simulink model "RedPrueba"  (R2015a)
settings: Solver=ode45  StartTime=0.0  StopTime=0.160  RelTol=1e-3
libraries: powerlib x20
settings Model: Creator=NECSOFT  LastModifiedBy=USUARIO

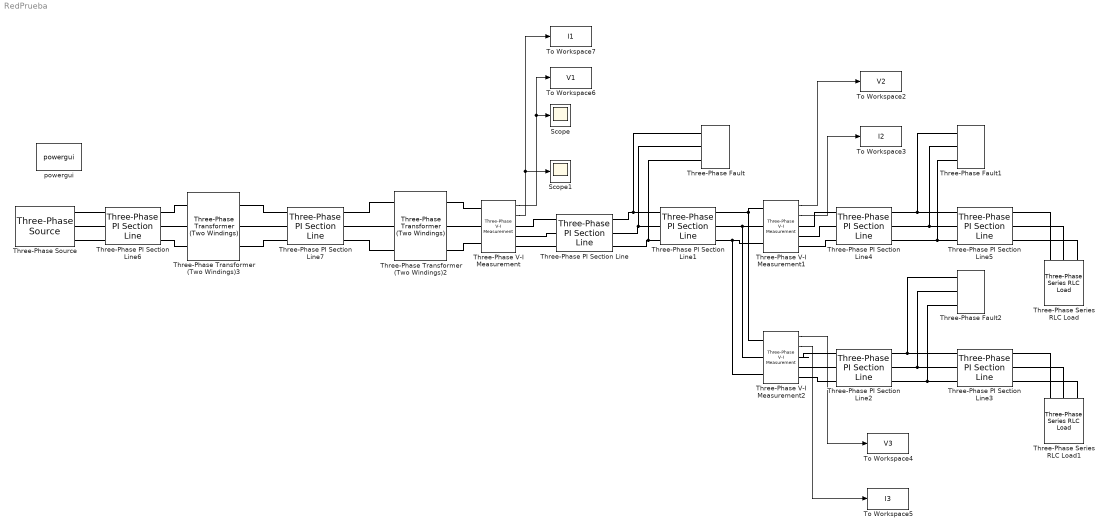
== system RedPrueba ==
  Scope : Scope
  Scope1 : Scope
  Three-Phase PI Section Line : powerlib/Elements/Three-Phase PI Section Line  LConnTagsString=a|b|c  RConnTagsString=A|B|C  Frequency=60  Resistances=[ 0.01273 0.3864]  Inductances="[ 0.9337e-3  4.1264e-3]"  Capacitances=[12.74e-9 7.751e-9]  Length=15
  Three-Phase PI Section Line1 : powerlib/Elements/Three-Phase PI Section Line  LConnTagsString=a|b|c  RConnTagsString=A|B|C  Frequency=60  Resistances=[ 0.01273 0.3864]  Inductances="[ 0.9337e-3  4.1264e-3]"  Capacitances=[12.74e-9 7.751e-9]  Length=5
  Three-Phase PI Section Line2 : powerlib/Elements/Three-Phase PI Section Line  LConnTagsString=a|b|c  RConnTagsString=A|B|C  Frequency=60  Resistances=[ 4*0.01273 4*0.3864]  Inductances="[ 4*0.9337e-3  4*4.1264e-3]"  Capacitances=[12.74e-9 7.751e-9]  Length=12
  Three-Phase PI Section Line3 : powerlib/Elements/Three-Phase PI Section Line  LConnTagsString=a|b|c  RConnTagsString=A|B|C  Frequency=60  Resistances=[ 4*0.01273 4*0.3864]  Inductances="[ 4*0.9337e-3  4*4.1264e-3]"  Capacitances=[12.74e-9 7.751e-9]  Length=8
  Three-Phase PI Section Line4 : powerlib/Elements/Three-Phase PI Section Line  LConnTagsString=a|b|c  RConnTagsString=A|B|C  Frequency=60  Resistances=[ 2*0.01273 2*0.3864]  Inductances="[ 2*0.9337e-3  2*4.1264e-3]"  Capacitances=[12.74e-9 7.751e-9]  Length=0.1
  Three-Phase PI Section Line5 : powerlib/Elements/Three-Phase PI Section Line  LConnTagsString=a|b|c  RConnTagsString=A|B|C  Frequency=60  Resistances=[ 2*0.01273 2*0.3864]  Inductances="[ 2*0.9337e-3  2*4.1264e-3]"  Capacitances=[12.74e-9 7.751e-9]  Length=19.9
  Three-Phase PI Section Line6 : powerlib/Elements/Three-Phase PI Section Line  LConnTagsString=a|b|c  RConnTagsString=A|B|C  Frequency=60  Resistances=[ 0.01273 0.3864]  Inductances="[ 0.9337e-3  4.1264e-3]"  Capacitances=[12.74e-9 7.751e-9]  Length=50
  Three-Phase PI Section Line7 : powerlib/Elements/Three-Phase PI Section Line  LConnTagsString=a|b|c  RConnTagsString=A|B|C  Frequency=60  Resistances=[ 0.01273 0.3864]  Inductances="[ 0.9337e-3  4.1264e-3]"  Capacitances=[12.74e-9 7.751e-9]  Length=100
  Three-Phase Series RLC Load : powerlib/Elements/Three-Phase Series RLC Load  LConnTagsString=A|B|C  Configuration=Y (grounded)  NominalVoltage=13800  NominalFrequency=60  ActivePower=100e3  InductivePower=0  CapacitivePower=0  Measurements=None  LoadType=constant Z
  Three-Phase Series RLC Load1 : powerlib/Elements/Three-Phase Series RLC Load  LConnTagsString=A|B|C  Configuration=Y (grounded)  NominalVoltage=13800  NominalFrequency=60  ActivePower=100e3  InductivePower=0  CapacitivePower=0  Measurements=None  LoadType=constant Z
  Three-Phase Transformer (Two Windings)2 : powerlib/Elements/Three-Phase Transformer (Two Windings)  Winding1Connection=Yg  Winding2Connection=Yg  CoreType=Three single-phase transformers  SetSaturation=off  Hysteresis=off  DataFile='hysteresis'  SetInitialFlux=off  Measurements=None  UNITS=pu  NominalPower=[ 5e6 , 60 ]  Winding1=[ 34500 , 0 , 0.0273 ]  Winding2=[ 13800 , 0 , 0.0273 ]  Rm=500  Lm=500  L0=0.5  Saturation=[ 0,0 ; 0.0024,1.2 ; 1.0,1.52 ]  InitialFluxes=[ 0.8 , -0.8 , 0.7 ]  MoreParameters=off  BreakLoop=off  DataType=off  TransfoNumber=1
  Three-Phase Transformer (Two Windings)3 : powerlib/Elements/Three-Phase Transformer (Two Windings)  Winding1Connection=Yg  Winding2Connection=Yg  CoreType=Three single-phase transformers  SetSaturation=off  Hysteresis=off  DataFile='hysteresis'  SetInitialFlux=off  Measurements=None  UNITS=pu  NominalPower=[ 40e6 , 60 ]  Winding1=[ 115000 , 0 , 0.06 ]  Winding2=[ 34500 , 0 , 0.06 ]  Rm=500  Lm=500  L0=0.5  Saturation=[ 0,0 ; 0.0024,1.2 ; 1.0,1.52 ]  InitialFluxes=[ 0.8 , -0.8 , 0.7 ]  MoreParameters=off  BreakLoop=off  DataType=off  TransfoNumber=1
  Three-Phase V-I Measurement : powerlib/Measurements/Three-Phase V-I Measurement  VoltageMeasurement=phase-to-ground  SetLabelV=off  LabelV=Vabc  Vpu=off  VpuLL=off  CurrentMeasurement=yes  SetLabelI=off  LabelI=Iabc  Ipu=off  Pbase=100e6  Vbase=500e3  OutputType=Complex  PhasorSimulation=off  PSBequivalent=0
  Three-Phase V-I Measurement1 : powerlib/Measurements/Three-Phase V-I Measurement  VoltageMeasurement=phase-to-ground  SetLabelV=off  LabelV=Vabc  Vpu=off  VpuLL=off  CurrentMeasurement=yes  SetLabelI=off  LabelI=Iabc  Ipu=off  Pbase=100e6  Vbase=500e3  OutputType=Complex  PhasorSimulation=off  PSBequivalent=0
  Three-Phase V-I Measurement2 : powerlib/Measurements/Three-Phase V-I Measurement  VoltageMeasurement=phase-to-ground  SetLabelV=off  LabelV=Vabc  Vpu=off  VpuLL=off  CurrentMeasurement=yes  SetLabelI=off  LabelI=Iabc  Ipu=off  Pbase=100e6  Vbase=500e3  OutputType=Complex  PhasorSimulation=off  PSBequivalent=0
  Three-Phase Fault : powerlib/Elements/Three-Phase Fault  InitialStates=0  FaultA=off  FaultB=off  FaultC=off  GroundFault=off  SwitchTimes="[3/60  6/60]"  External=off  SwitchStatus=NaN  FaultResistance=0.001  GroundResistance=0.01  SnubberResistance=1e6  SnubberCapacitance=inf  Measurements=None
  Three-Phase Fault1 : powerlib/Elements/Three-Phase Fault  InitialStates=0  FaultA=off  FaultB=on  FaultC=off  GroundFault=on  SwitchTimes="[2/60  6/60]"  External=off  SwitchStatus=NaN  FaultResistance=1  GroundResistance=0.01  SnubberResistance=1e6  SnubberCapacitance=inf  Measurements=None
  Three-Phase Fault2 : powerlib/Elements/Three-Phase Fault  InitialStates=0  FaultA=off  FaultB=off  FaultC=off  GroundFault=off  SwitchTimes="[6/60  8/60]"  External=off  SwitchStatus=NaN  FaultResistance=0.001  GroundResistance=0.01  SnubberResistance=1e6  SnubberCapacitance=inf  Measurements=None
  Three-Phase Source : powerlib/Electrical Sources/Three-Phase Source  Voltage=115000  PhaseAngle=0  Frequency=60  InternalConnection=Yg  SpecifyImpedance=on  Resistance=0.8929  Inductance=16.58e-3  ShortCircuitLevel=100e6  BaseVoltage=13.2e3  XRratio=7  BusType=swing  Pref=0  Qref=0  Qmin=-inf  Qmax=inf
  To Workspace2 : ToWorkspace  VariableName=V2  SampleTime=-1
  To Workspace3 : ToWorkspace  VariableName=I2  SampleTime=-1
  To Workspace4 : ToWorkspace  VariableName=V3  SampleTime=-1
  To Workspace5 : ToWorkspace  VariableName=I3  SampleTime=-1
  To Workspace6 : ToWorkspace  VariableName=V1  SampleTime=-1
  To Workspace7 : ToWorkspace  VariableName=I1  SampleTime=-1
  powergui : powerlib/powergui  Priority=1  SimulationMode=Discrete  SolverType=Tustin/Backward Euler (TBE)  SampleTime=1/(32*60)  frequency=60  SPID=off  DisableSnubberDevices=off  DisableRonSwitches=off  DisableVfSwitches=off  SwTol=0  DisplayEquations=off  Interpol=off  methode=off  Ts=100  FunctionMessages=off  echomessages=off  HookPort=off  EnableUseOfTLC=off  x0status=blocks  frequencyindice=0  Pbase=100e6  ErrMax=1e-4  Iterations=50  UnitsV=kV  UnitsW=MW  buscounter=0  RestoreLinks=warning  ResistiveCurrentMeasurement=off  Frange=[0:2:500]  Ylog=off  Xlog=on  ShowGrid=off  save=off  variable=ZData  structure=0  ZoomFFT=off  StartTime=0.0  cycles=1  DisplayStyle=1  fundamental=60  FreqAxis=off  MaxFrequency=1000  frequencyindicesteady=1  RmsSteady=1  display=off
  wires:
  Three-Phase V-I Measurement/1 -> To Workspace6/1, Scope/1
  Three-Phase V-I Measurement/2 -> To Workspace7/1, Scope1/1
  Three-Phase V-I Measurement1/1 -> To Workspace2/1
  Three-Phase V-I Measurement1/2 -> To Workspace3/1
  Three-Phase V-I Measurement2/1 -> To Workspace4/1
  Three-Phase V-I Measurement2/2 -> To Workspace5/1
  connections:
  Three-Phase PI Section Line1/LConn3 -- Three-Phase Fault/LConn3 -- Three-Phase PI Section Line/RConn3
  Three-Phase PI Section Line1/LConn2 -- Three-Phase Fault/LConn2 -- Three-Phase PI Section Line/RConn2
  Three-Phase PI Section Line1/LConn1 -- Three-Phase Fault/LConn1 -- Three-Phase PI Section Line/RConn1
  Three-Phase PI Section Line3/LConn1 -- Three-Phase Fault2/LConn1 -- Three-Phase PI Section Line2/RConn1
  Three-Phase PI Section Line3/LConn2 -- Three-Phase Fault2/LConn2 -- Three-Phase PI Section Line2/RConn2
  Three-Phase PI Section Line3/LConn3 -- Three-Phase Fault2/LConn3 -- Three-Phase PI Section Line2/RConn3
  Three-Phase PI Section Line5/LConn1 -- Three-Phase Fault1/LConn1 -- Three-Phase PI Section Line4/RConn1
  Three-Phase PI Section Line5/LConn2 -- Three-Phase Fault1/LConn2 -- Three-Phase PI Section Line4/RConn2
  Three-Phase PI Section Line5/LConn3 -- Three-Phase Fault1/LConn3 -- Three-Phase PI Section Line4/RConn3
  Three-Phase PI Section Line5/RConn1 -- Three-Phase Series RLC Load/LConn1
  Three-Phase PI Section Line5/RConn2 -- Three-Phase Series RLC Load/LConn2
  Three-Phase PI Section Line5/RConn3 -- Three-Phase Series RLC Load/LConn3
  Three-Phase PI Section Line3/RConn1 -- Three-Phase Series RLC Load1/LConn1
  Three-Phase PI Section Line3/RConn2 -- Three-Phase Series RLC Load1/LConn2
  Three-Phase PI Section Line3/RConn3 -- Three-Phase Series RLC Load1/LConn3
  Three-Phase PI Section Line6/LConn1 -- Three-Phase Source/RConn1
  Three-Phase PI Section Line6/LConn2 -- Three-Phase Source/RConn2
  Three-Phase PI Section Line6/LConn3 -- Three-Phase Source/RConn3
  Three-Phase V-I Measurement/RConn1 -- Three-Phase PI Section Line/LConn1
  Three-Phase V-I Measurement/RConn2 -- Three-Phase PI Section Line/LConn2
  Three-Phase V-I Measurement/RConn3 -- Three-Phase PI Section Line/LConn3
  Three-Phase PI Section Line1/RConn1 -- Three-Phase V-I Measurement2/LConn1 -- Three-Phase V-I Measurement1/LConn1
  Three-Phase PI Section Line1/RConn2 -- Three-Phase V-I Measurement2/LConn2 -- Three-Phase V-I Measurement1/LConn2
  Three-Phase PI Section Line1/RConn3 -- Three-Phase V-I Measurement2/LConn3 -- Three-Phase V-I Measurement1/LConn3
  Three-Phase V-I Measurement1/RConn1 -- Three-Phase PI Section Line4/LConn1
  Three-Phase V-I Measurement1/RConn2 -- Three-Phase PI Section Line4/LConn2
  Three-Phase V-I Measurement1/RConn3 -- Three-Phase PI Section Line4/LConn3
  Three-Phase V-I Measurement2/RConn1 -- Three-Phase PI Section Line2/LConn1
  Three-Phase V-I Measurement2/RConn2 -- Three-Phase PI Section Line2/LConn2
  Three-Phase V-I Measurement2/RConn3 -- Three-Phase PI Section Line2/LConn3
  Three-Phase PI Section Line6/RConn1 -- Three-Phase Transformer (Two Windings)3/LConn1
  Three-Phase PI Section Line6/RConn2 -- Three-Phase Transformer (Two Windings)3/LConn2
  Three-Phase PI Section Line6/RConn3 -- Three-Phase Transformer (Two Windings)3/LConn3
  Three-Phase Transformer (Two Windings)3/RConn1 -- Three-Phase PI Section Line7/LConn1
  Three-Phase Transformer (Two Windings)3/RConn2 -- Three-Phase PI Section Line7/LConn2
  Three-Phase Transformer (Two Windings)3/RConn3 -- Three-Phase PI Section Line7/LConn3
  Three-Phase PI Section Line7/RConn1 -- Three-Phase Transformer (Two Windings)2/LConn1
  Three-Phase PI Section Line7/RConn2 -- Three-Phase Transformer (Two Windings)2/LConn2
  Three-Phase PI Section Line7/RConn3 -- Three-Phase Transformer (Two Windings)2/LConn3
  Three-Phase Transformer (Two Windings)2/RConn1 -- Three-Phase V-I Measurement/LConn1
  Three-Phase Transformer (Two Windings)2/RConn2 -- Three-Phase V-I Measurement/LConn2
  Three-Phase Transformer (Two Windings)2/RConn3 -- Three-Phase V-I Measurement/LConn3
